simulink model "augment_integrator"  (R2022a)
settings: Solver=VariableStepAuto  StartTime=0.0  StopTime=10.0  RelTol=1e-3
values from neighbouring files (symbols this model uses):
  A = [0 1;0 3]    [aug_int.m]
  B = [0; 1]    [aug_int.m]
  C = [1 1]    [aug_int.m]
  G = [-2 -2]    [aug_int.m]
  K = [-1; 5]    [aug_int.m]
  sigma_y = 1    [aug_int.m]
settings Model: Creator=Tris  LastModifiedBy=Tris

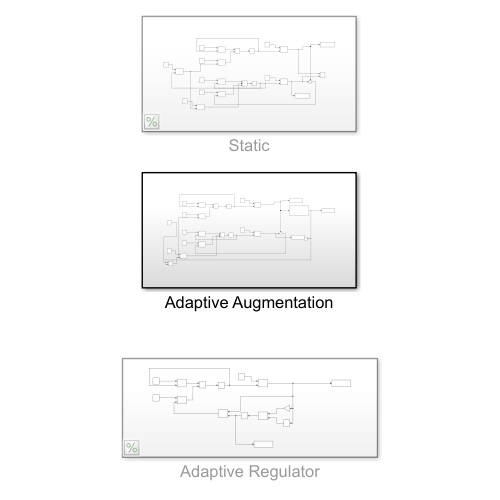
[thumbnail: Simulink's stored preview of the top-level diagram]
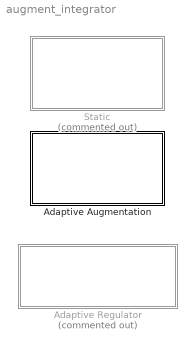
== system augment_integrator ==
  Adaptive Augmentation : Subsystem
  Adaptive Regulator : Subsystem  Commented=on
  Static : Subsystem  Commented=on

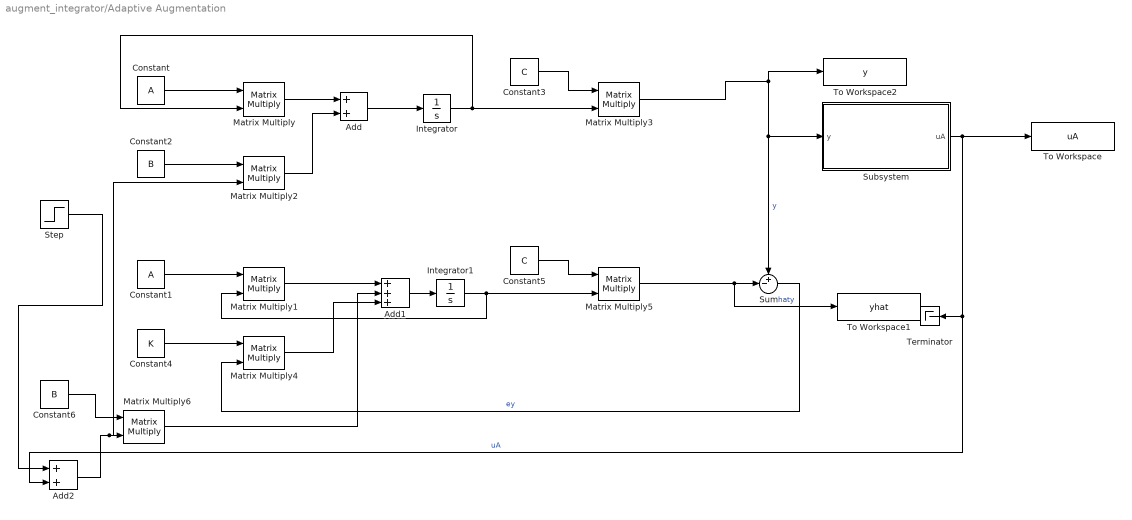
== system augment_integrator/Adaptive Augmentation ==
  Add : Sum
  Add1 : Sum  Inputs=+++
  Add2 : Sum
  Constant : Constant  Value=A  VectorParams1D=off
  Constant1 : Constant  Value=A  VectorParams1D=off
  Constant2 : Constant  Value=B  VectorParams1D=off
  Constant3 : Constant  Value=C  VectorParams1D=off
  Constant4 : Constant  Value=K  VectorParams1D=off
  Constant5 : Constant  Value=C  VectorParams1D=off
  Constant6 : Constant  Value=B  VectorParams1D=off
  Integrator : Integrator  InitialCondition=[1; -1]
  Integrator1 : Integrator  InitialCondition=[-1; 1]
  Matrix Multiply{,1..6} (7 alike) : Product  Multiplication=Matrix(*)
  Step : Step  SampleTime=0
  Subsystem : Subsystem
  Sum : Sum  Inputs=+-|
  Terminator : Terminator
  To Workspace : ToWorkspace  VariableName=uA  SaveFormat=Timeseries  SampleTime=-1
  To Workspace1 : ToWorkspace  VariableName=yhat  SaveFormat=Timeseries  SampleTime=-1
  To Workspace2 : ToWorkspace  VariableName=y  SaveFormat=Timeseries  SampleTime=-1
  wires:
  Subsystem/1(uA) -> To Workspace/1, Add2/2, Terminator/1  "uA"
  Integrator/1 -> Matrix Multiply3/2, Matrix Multiply/2
  Matrix Multiply3/1 -> Sum/1, Subsystem/1(y), To Workspace2/1  "y"
  Constant6/1 -> Matrix Multiply6/1
  Add1/1 -> Integrator1/1
  Integrator1/1 -> Matrix Multiply5/2, Matrix Multiply1/2
  Matrix Multiply2/1 -> Add/2
  Add2/1 -> Matrix Multiply2/2, Matrix Multiply6/2
  Matrix Multiply5/1 -> To Workspace1/1, Sum/2  "haty"
  Constant3/1 -> Matrix Multiply3/1
  Matrix Multiply1/1 -> Add1/1
  Add/1 -> Integrator/1
  Matrix Multiply6/1 -> Add1/2
  Constant/1 -> Matrix Multiply/1
  Constant5/1 -> Matrix Multiply5/1
  Constant4/1 -> Matrix Multiply4/1
  Constant1/1 -> Matrix Multiply1/1
  Matrix Multiply/1 -> Add/1
  Step/1 -> Add2/1
  Sum/1 -> Matrix Multiply4/2  "ey"
  Constant2/1 -> Matrix Multiply2/1
  Matrix Multiply4/1 -> Add1/3

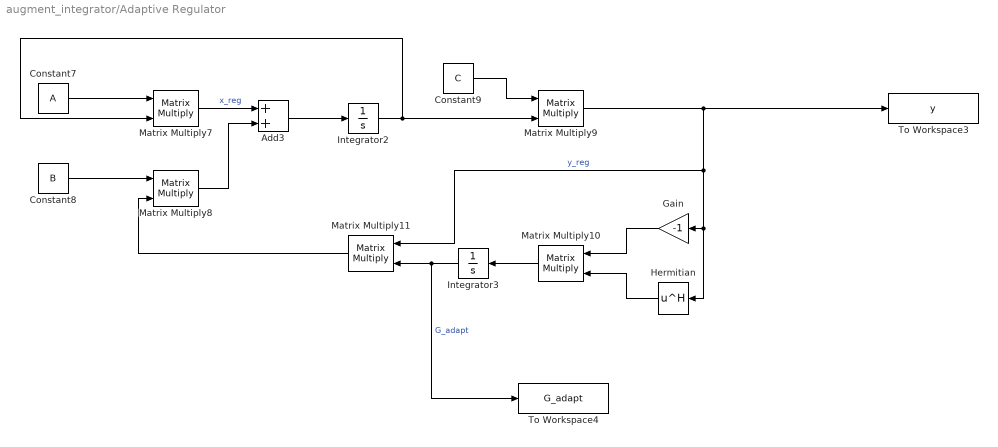
== system augment_integrator/Adaptive Regulator ==
  Add3 : Sum
  Constant7 : Constant  Value=A  VectorParams1D=off
  Constant8 : Constant  Value=B  VectorParams1D=off
  Constant9 : Constant  Value=C  VectorParams1D=off
  Gain : Gain  Gain=-1
  Hermitian : Math  Operator=hermitian
  Integrator2 : Integrator  InitialCondition=[1; -1]
  Integrator3 : Integrator
  Matrix Multiply{7..11} (5 alike) : Product  Multiplication=Matrix(*)
  To Workspace3 : ToWorkspace  VariableName=y  SaveFormat=Timeseries  SampleTime=-1
  To Workspace4 : ToWorkspace  VariableName=G_adapt  SaveFormat=Timeseries  SampleTime=-1
  wires:
  Integrator2/1 -> Matrix Multiply9/2, Matrix Multiply7/2
  Constant7/1 -> Matrix Multiply7/1
  Matrix Multiply7/1 -> Add3/1  "x_reg"
  Constant9/1 -> Matrix Multiply9/1
  Constant8/1 -> Matrix Multiply8/1
  Add3/1 -> Integrator2/1
  Matrix Multiply10/1 -> Integrator3/1
  Matrix Multiply8/1 -> Add3/2
  Matrix Multiply9/1 -> To Workspace3/1, Matrix Multiply11/1, Hermitian/1, Gain/1  "y_reg"
  Hermitian/1 -> Matrix Multiply10/2
  Gain/1 -> Matrix Multiply10/1
  Integrator3/1 -> To Workspace4/1, Matrix Multiply11/2  "G_adapt"
  Matrix Multiply11/1 -> Matrix Multiply8/2

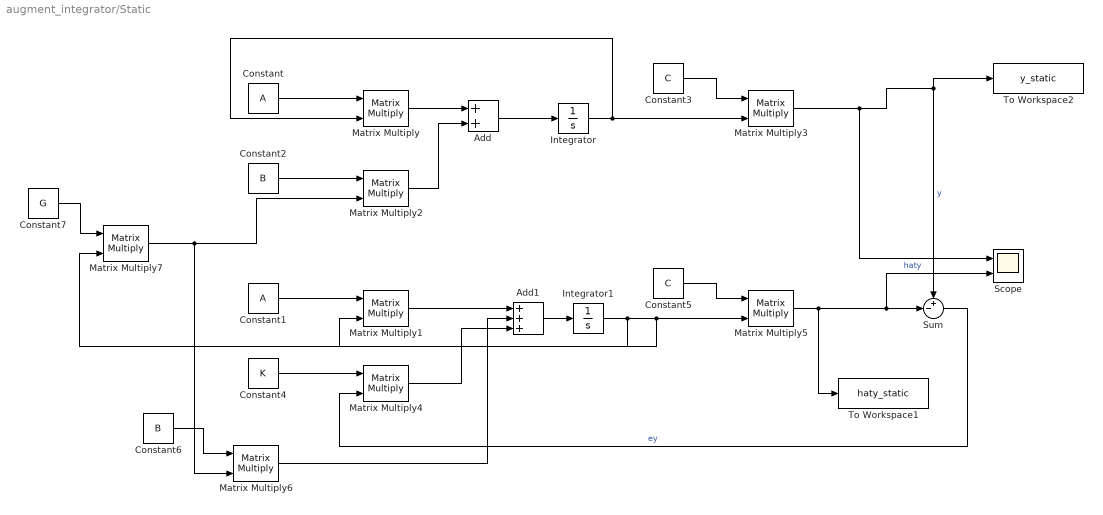
== system augment_integrator/Static ==
  Add : Sum
  Add1 : Sum  Inputs=+++
  Constant : Constant  Value=A  VectorParams1D=off
  Constant1 : Constant  Value=A  VectorParams1D=off
  Constant2 : Constant  Value=B  VectorParams1D=off
  Constant3 : Constant  Value=C  VectorParams1D=off
  Constant4 : Constant  Value=K  VectorParams1D=off
  Constant5 : Constant  Value=C  VectorParams1D=off
  Constant6 : Constant  Value=B  VectorParams1D=off
  Constant7 : Constant  Value=G  VectorParams1D=off
  Integrator : Integrator  InitialCondition=[1; -1]
  Integrator1 : Integrator  InitialCondition=[-1; 1]
  Matrix Multiply{,1..7} (8 alike) : Product  Multiplication=Matrix(*)
  Scope : Scope  NumInputPorts=2
  Sum : Sum  Inputs=+-|
  To Workspace1 : ToWorkspace  VariableName=haty_static  SaveFormat=Timeseries  SampleTime=-1
  To Workspace2 : ToWorkspace  VariableName=y_static  SaveFormat=Timeseries  SampleTime=-1
  wires:
  Integrator/1 -> Matrix Multiply3/2, Matrix Multiply/2
  Matrix Multiply3/1 -> Scope/1, Sum/1, To Workspace2/1  "y"
  Constant6/1 -> Matrix Multiply6/1
  Add1/1 -> Integrator1/1
  Integrator1/1 -> Matrix Multiply7/2, Matrix Multiply5/2, Matrix Multiply1/2
  Matrix Multiply2/1 -> Add/2
  Matrix Multiply5/1 -> To Workspace1/1, Scope/2, Sum/2  "haty"
  Constant3/1 -> Matrix Multiply3/1
  Matrix Multiply1/1 -> Add1/1
  Add/1 -> Integrator/1
  Matrix Multiply6/1 -> Add1/2
  Constant/1 -> Matrix Multiply/1
  Constant5/1 -> Matrix Multiply5/1
  Constant4/1 -> Matrix Multiply4/1
  Constant1/1 -> Matrix Multiply1/1
  Matrix Multiply/1 -> Add/1
  Sum/1 -> Matrix Multiply4/2  "ey"
  Constant2/1 -> Matrix Multiply2/1
  Matrix Multiply4/1 -> Add1/3
  Matrix Multiply7/1 -> Matrix Multiply6/2, Matrix Multiply2/2
  Constant7/1 -> Matrix Multiply7/1

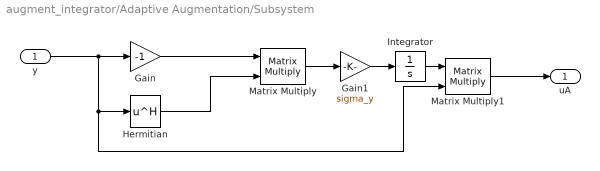
== system augment_integrator/Adaptive Augmentation/Subsystem ==
  y : Inport
  Gain : Gain  Gain=-1
  Gain1 : Gain  Gain=sigma_y
  Hermitian : Math  Operator=hermitian
  Integrator : Integrator
  Matrix Multiply : Product  Multiplication=Matrix(*)
  Matrix Multiply1 : Product  Multiplication=Matrix(*)
  uA : Outport
  wires:
  y/1 -> Matrix Multiply1/2, Hermitian/1, Gain/1
  Gain/1 -> Matrix Multiply/1
  Hermitian/1 -> Matrix Multiply/2
  Matrix Multiply/1 -> Gain1/1
  Gain1/1 -> Integrator/1
  Matrix Multiply1/1 -> uA/1
  Integrator/1 -> Matrix Multiply1/1
